simulink model "simulink_test1"  (R2019a)
settings: Solver=VariableStepAuto  StartTime=0.0  StopTime=10.0  RelTol=1e-3
libraries: simulink x3
settings Model: Creator=rosha  LastModifiedBy=rosha

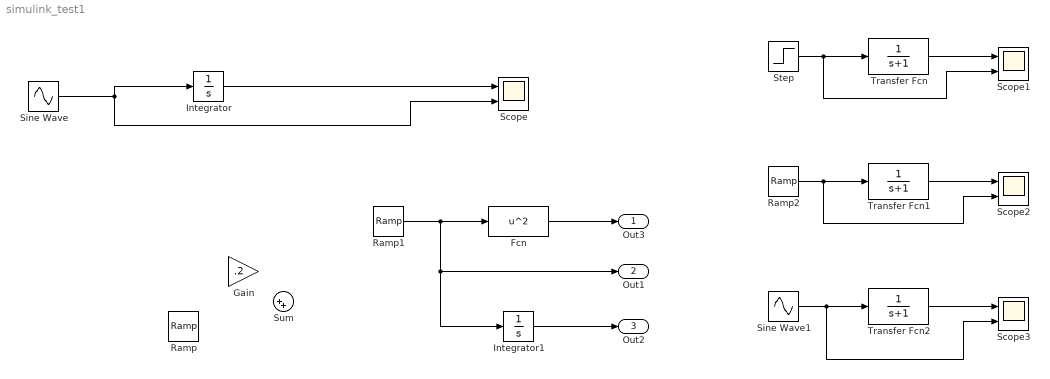
== system simulink_test1 ==
  Fcn : Fcn  Expr=u^2
  Gain : Gain  Gain=.2
  Integrator : Integrator
  Integrator1 : Integrator
  Ramp : simulink/Sources/Ramp  slope=1  start=0  InitialOutput=0
  Ramp1 : simulink/Sources/Ramp  slope=1  start=0  InitialOutput=0
  Ramp2 : simulink/Sources/Ramp  slope=1  start=0  InitialOutput=0
  Scope{,1..3} (4 alike) : Scope  NumInputPorts=2
  Sine Wave : Sin  SampleTime=0
  Sine Wave1 : Sin  SampleTime=0
  Step : Step  SampleTime=0
  Sum : Sum  Inputs=|++
  Transfer Fcn : TransferFcn  Denominator=[1 1]
  Transfer Fcn1 : TransferFcn  Denominator=[1 1]
  Transfer Fcn2 : TransferFcn  Denominator=[1 1]
  Out3 : Outport
  Out1 : Outport  Port=2
  Out2 : Outport  Port=3
  wires:
  Integrator/1 -> Scope/1
  Sine Wave/1 -> Integrator/1, Scope/2
  Fcn/1 -> Out3/1
  Ramp1/1 -> Integrator1/1, Out1/1, Fcn/1
  Integrator1/1 -> Out2/1
  Step/1 -> Scope1/2, Transfer Fcn/1
  Transfer Fcn/1 -> Scope1/1
  Transfer Fcn1/1 -> Scope2/1
  Ramp2/1 -> Scope2/2, Transfer Fcn1/1
  Sine Wave1/1 -> Transfer Fcn2/1, Scope3/2
  Transfer Fcn2/1 -> Scope3/1
